simulink model "Direct_Force_Pose_NMPC_Practice"  (R2021a)
settings: Solver=VariableStepAuto  StartTime=0.0  StopTime=5  RelTol=1e-3
libraries: simulink x1, mpclib x1
settings Model: Creator=Hameed  LastModifiedBy=Hameed

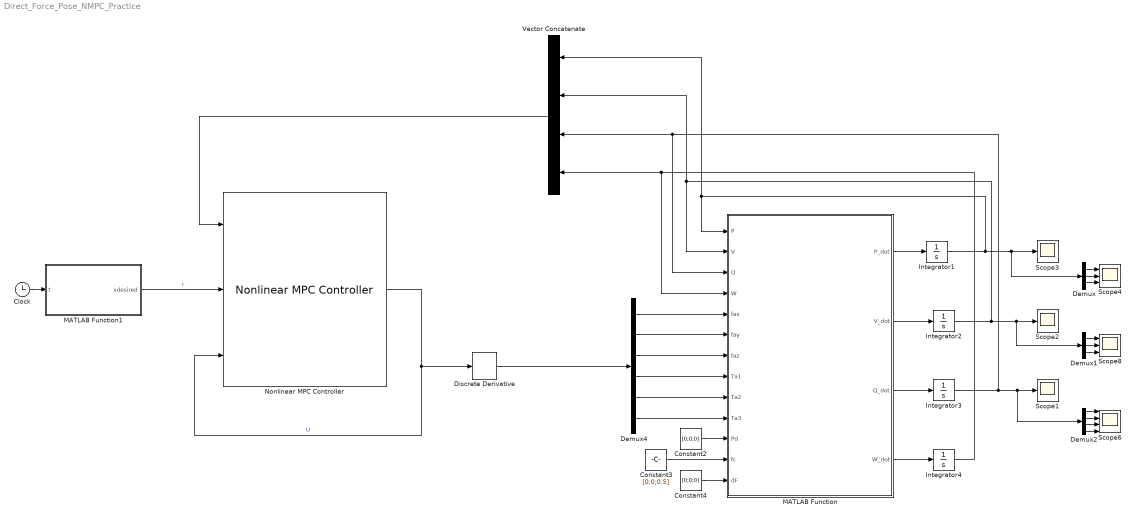
== system Direct_Force_Pose_NMPC_Practice ==
  Clock : Clock
  Constant2 : Constant  Value=[0;0;0]  VectorParams1D=off
  Constant3 : Constant  Value=[0;0;0.5]  VectorParams1D=off
  Constant4 : Constant  Value=[0;0;0]  VectorParams1D=off
  Demux : Demux  Outputs=3
  Demux1 : Demux  Outputs=3
  Demux2 : Demux
  Demux4 : Demux  Outputs=6
  Discrete Derivative : simulink/Discrete/Discrete Derivative  gainval=1.0  ICPrevScaledInput=0.0  OutMin=[]  OutMax=[]  OutDataType=fixdt(1, 16)  OutScaling=2^-10  DoSatur=off
  Integrator1 : Integrator  InitialCondition=[0;0;0]
  Integrator2 : Integrator  InitialCondition=[0;0;0]
  Integrator3 : Integrator  InitialCondition=[0;0;0;0]
  Integrator4 : Integrator  InitialCondition=[0;0;0]
  MATLAB Function : MATLAB Function  TreatAsAtomicUnit=on
  MATLAB Function1 : MATLAB Function  TreatAsAtomicUnit=on
  Nonlinear MPC Controller : mpclib/Nonlinear MPC Controller  SCDEnableBlockLinearizationSpecification=on  nlmpcobj=nlobj  UseObjectTs=on  UseMEX=off  md_enabled=off  mvtarget_enabled=off  param_enabled=off  cost_enabled=off  mvseq_enabled=off  stateseq_enabled=off  ovseq_enabled=off  slack_enabled=off  status_enabled=off  ov_min=off  ov_max=off  mv_min=off  mv_max=off  mvrate_min=off  mvrate_max=off  state_min=off  state_max=off  ov_weight=off  mv_weight=off  mvrate_weight=off  ecr_weight=off  nlp_initialize=off
  Scope1 : Scope
  Scope2 : Scope
  Scope3 : Scope
  Scope4 : Scope  NumInputPorts=3
  Scope6 : Scope  NumInputPorts=4
  Scope8 : Scope  NumInputPorts=3
  Vector Concatenate : Concatenate  NumInputs=4
  wires:
  Constant4/1 -> MATLAB Function/13(dF)
  MATLAB Function/2(V_dot) -> Integrator2/1
  Constant2/1 -> MATLAB Function/11(Pd)
  Integrator2/1 -> MATLAB Function/2(V), Vector Concatenate/2, Scope2/1, Demux1/1
  MATLAB Function/3(Q_dot) -> Integrator3/1
  Integrator4/1 -> MATLAB Function/4(W), Vector Concatenate/4
  MATLAB Function/1(P_dot) -> Integrator1/1
  Constant3/1 -> MATLAB Function/12(fc)
  Integrator1/1 -> MATLAB Function/1(P), Vector Concatenate/1, Scope3/1, Demux/1
  MATLAB Function/4(W_dot) -> Integrator4/1
  Demux/1 -> Scope4/1
  Demux/2 -> Scope4/2
  Demux/3 -> Scope4/3
  Demux1/3 -> Scope8/3
  Demux1/1 -> Scope8/1
  Demux1/2 -> Scope8/2
  Demux2/3 -> Scope6/3
  Demux2/2 -> Scope6/2
  Demux2/1 -> Scope6/1
  Integrator3/1 -> MATLAB Function/3(Q), Vector Concatenate/3, Scope1/1, Demux2/1
  Demux2/4 -> Scope6/4
  Nonlinear MPC Controller/1 -> Nonlinear MPC Controller/3, Discrete Derivative/1  "U"
  Vector Concatenate/1 -> Nonlinear MPC Controller/1
  Clock/1 -> MATLAB Function1/1(t)
  MATLAB Function1/1(xdesired) -> Nonlinear MPC Controller/2  "r"
  Demux4/1 -> MATLAB Function/5(fax)
  Demux4/2 -> MATLAB Function/6(fay)
  Demux4/3 -> MATLAB Function/7(faz)
  Demux4/4 -> MATLAB Function/8(Ta1)
  Demux4/5 -> MATLAB Function/9(Ta2)
  Demux4/6 -> MATLAB Function/10(Ta3)
  Discrete Derivative/1 -> Demux4/1

== matlab function Direct_Force_Pose_NMPC_Practice/MATLAB Function1 ==
  data: t input; xdesired output
function xdesired   = multirotorReferenceTrajectory( t )
% This function generates reference signal for nonlinear MPC controller
% used in the quadrotor path following example.

% Copyright 2019 The MathWorks, Inc.

%#codegen
x =0.5*sin(t/3);
y = -0.5*sin(t/3).*cos(t/3);
z = 0.5*cos(t/3);
%z = 10+zeros(1,length(t));
zero=zeros(1,length(t));
% phi = zeros(1,length(t));
% theta = zeros(1,length(t));
% psi = zeros(1,length(t));
phi = pi/6*sin(t/3);
theta = -pi/3*sin(t/3).*cos(t/3);
psi = pi*ones(1,length(t));

xdot = zeros(1,length(t));
ydot = zeros(1,length(t));
zdot = zeros(1,length(t));
phidot = zeros(1,length(t));
thetadot = zeros(1,length(t));
psidot = zeros(1,length(t));

xdesired = [x;y;z; zero; phi;theta;psi;xdot;ydot;zdot;phidot;thetadot;psidot]';
end

== matlab function Direct_Force_Pose_NMPC_Practice/MATLAB Function ==
  data: P input; P_dot output; V input; Q input; W input; V_dot output; Q_dot output; W_dot output; fax input; fay input; faz input; Ta1 input; Ta2 input; Ta3 input; Pd input; fc input; dF input
function [P_dot,V_dot,Q_dot,W_dot]= fcn(P,V,Q,W,fax,fay,faz,Ta1,Ta2,Ta3,Pd,fc,dF)
clc
m=5;

% theta=Q(2);
% phi=Q(3);
% psi=Q(4);

% Rz=[cos(psi) sin(psi) 0;-sin(psi)) cos(psi) 0;0 0 1];
% Rx=[1 0 0;0 cos(theta) sin(theta);0 -sin(theta) cos(theta)];
% Ry=[cos(phi) 0 sin(phi);0 1 0;-sin(phi) 0 cos(phi)];

Rz=[cos(Q(4)) sin(Q(4)) 0;-sin(Q(4)) cos(Q(4)) 0;0 0 1];
Rx=[1 0 0;0 cos(Q(2)) sin(Q(2));0 -sin(Q(2)) cos(Q(2))];
Ry=[cos(Q(3)) 0 sin(Q(3));0 1 0;-sin(Q(3)) 0 cos(Q(3))];

%Rs=Rz*Rx*Ry;
Rs=[1 0 0;0 -1 0;0 0 -1];
%lambda=L;
L=0;
%L=1;
Rd=[1 0 0;0 1 0;0 0 1-L];
SL=Rs*Rd*transpose(Rs);
%V=[Vx;Vy;Vz];
%Rb=Rz;
Rb=[1 0 0;0 1 0;0 0 1];
%Rd=[1 0 0;0 1 0;0 0 1];
%fa=[fax;fay;faz];

P_dot=SL*V;
%rT=[rx;ry;rz];
%rT=P-Pd;
rT=[0.5;0;0];
%W=[Wx;Wy;Wz];

Q_dot=(1/2)*Q.*[0;W];

g=9.8;
%dF=[0;0;0.5];
dF=[0;0;0];
fc=[0;0;0.5];
%F=L*fc; as L=1
%F=fc;

% fax=fa(1);
% fay=fa(1);
% faz=fa(1);
% fa=[fax;fay;faz];
fa=[fax;fay;faz];
%fa=[fa(1);fa(2);fa(3)];
ab=(m^-1)*((Rb*fa)+(L*fc)+dF)+[0;0;g];

Ixx=1;
Iyy=1;
Izz=1;
J=[Ixx 0 0;0 Iyy 0;0 0 Izz];

%ta=[tx;ty;tz];
ta=[Ta1;Ta2;Ta3];

h=J*W;
rcom=[0;0;0];
%rcom=[0.05;0.05;0.05];
h1=transpose(Rb)*[0;0;m*g];
dT=[0;0;0];
%dT=[2;2;2];
h2=L*transpose(Rb)*fc;

W_dot=(inv(J))*(ta-cross(W,h)+cross(rcom,h1)+cross(rT,h2)+dT);

%ab=(m^-1)*((Rb*fa)+(L*fc)+dF)+[0;0;g];

V_dot=SL*((ab)+Rb*(cross(W_dot,rT)+(cross(W,cross(W,rT)))));
